simulink model "ForwardKinematicsModel"  (R2024b)
settings: Solver=VariableStepAuto  StartTime=0.0  StopTime=10.0  RelTol=1e-3
settings Model: Creator=pinto  LastModifiedBy=pinto

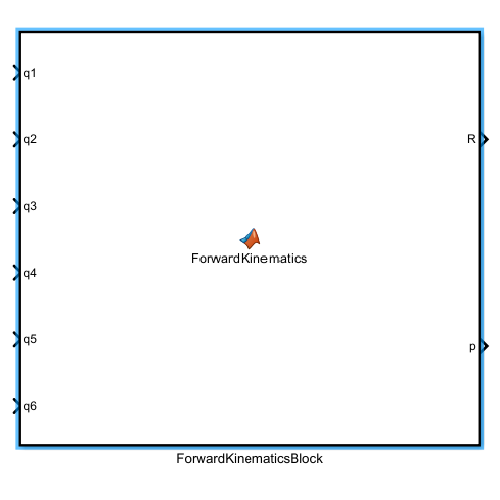
[thumbnail: Simulink's stored preview of the top-level diagram]
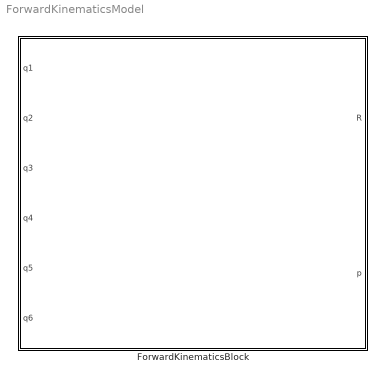
== system ForwardKinematicsModel ==
  ForwardKinematicsBlock : MATLAB Function  TreatAsAtomicUnit=on

== matlab function ForwardKinematicsModel/ForwardKinematicsBlock ==
  data: q1 input; R output; q2 input; q3 input; q4 input; q5 input; q6 input; p output
function [R, p] = ForwardKinematics(q1, q2, q3, q4, q5, q6)
% Entradas: q1...q6 (ângulos das juntas em rad)
% Saídas:
%   R - matriz de rotação 3x3
%   p - vetor posição 3x1

% Parâmetros DH: [d, theta, a, alpha, offset]
DH = [ 0     q1  0     pi/2      pi/2;
       0     q2  0    -pi/2      pi/2;
       0.4   q3  0     pi/2      pi/2;
       0     q4  0.1   pi/2     -pi/2;
       0.5   q5  0    -pi/2      0;
       0.1   q6  0     pi/2-pi/8 -pi/2;
       0.15  0   0     0         0 ];

T = eye(4);
for i = 1:size(DH,1)
    d = DH(i,1);
    theta = DH(i,2) + DH(i,5);
    a = DH(i,3);
    alpha = DH(i,4);

    A = [ cos(theta), -sin(theta)*cos(alpha),  sin(theta)*sin(alpha), a*cos(theta);
          sin(theta),  cos(theta)*cos(alpha), -cos(theta)*sin(alpha), a*sin(theta);
          0,           sin(alpha),             cos(alpha),            d;
          0,           0,                      0,                     1 ];

    T = T * A;
end

R = T(1:3, 1:3);
p = T(1:3, 4);
